simulink model "add_divide_multiply"  (R2024b)
settings: Solver=VariableStepAuto  StartTime=0.0  StopTime=10.0  RelTol=1e-3
settings Model: Creator=optimus  LastModifiedBy=optimus

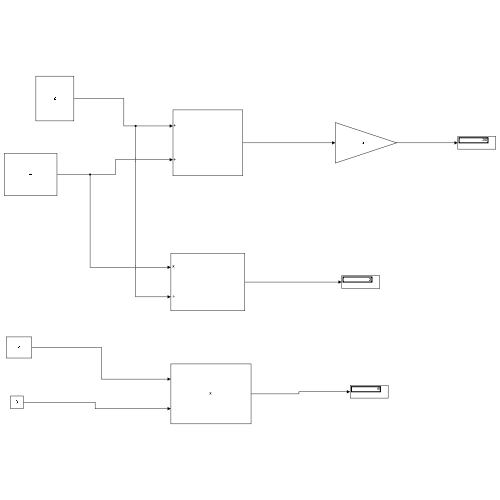
[thumbnail: Simulink's stored preview of the top-level diagram]
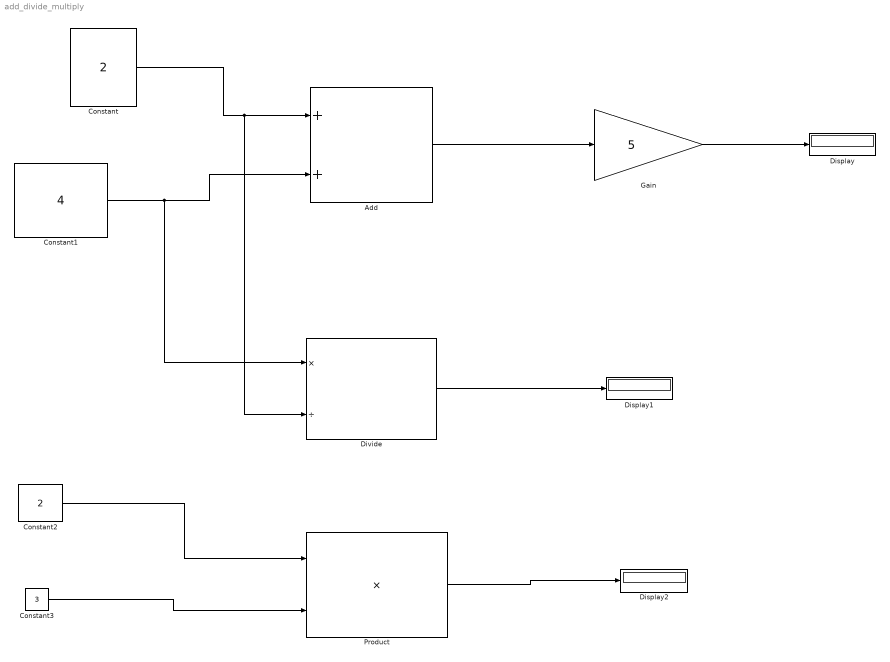
== system add_divide_multiply ==
  Add : Sum
  Constant : Constant  Value=2
  Constant1 : Constant  Value=4
  Constant2 : Constant  Value=2
  Constant3 : Constant  Value=3
  Display : Display
  Display1 : Display
  Display2 : Display
  Divide : Product  Inputs=*/
  Gain : Gain  Gain=5
  Product : Product
  wires:
  Constant/1 -> Divide/2, Add/1
  Constant1/1 -> Divide/1, Add/2
  Add/1 -> Gain/1
  Gain/1 -> Display/1
  Divide/1 -> Display1/1
  Constant2/1 -> Product/1
  Constant3/1 -> Product/2
  Product/1 -> Display2/1
